simulink model "CTModel"  (R2021a)
settings: Solver=ode4  StartTime=0.0  StopTime=tstop  FixedStep=tstep  RelTol=1e-3
values from neighbouring files (symbols this model uses):
  ldotic = [-0.001; 0.005]    [data.m]
  Vmic = 1000    [data.m]
  xic = [15000; -30*d2r; 45*d2r; 10*d2r; 10*d2r; 20*d2r; 135*d2r]    [data.m]
settings Model: Creator=Ram Padmanabhan  LastModifiedBy=Ram Padmanabhan
settings DataIOCC: SaveOutput=off  SignalLogging=off  DSMLogging=off  SaveTime=off  ReturnWorkspaceOutputs=off
settings DebuggingCC: AlgebraicLoopMsg=none

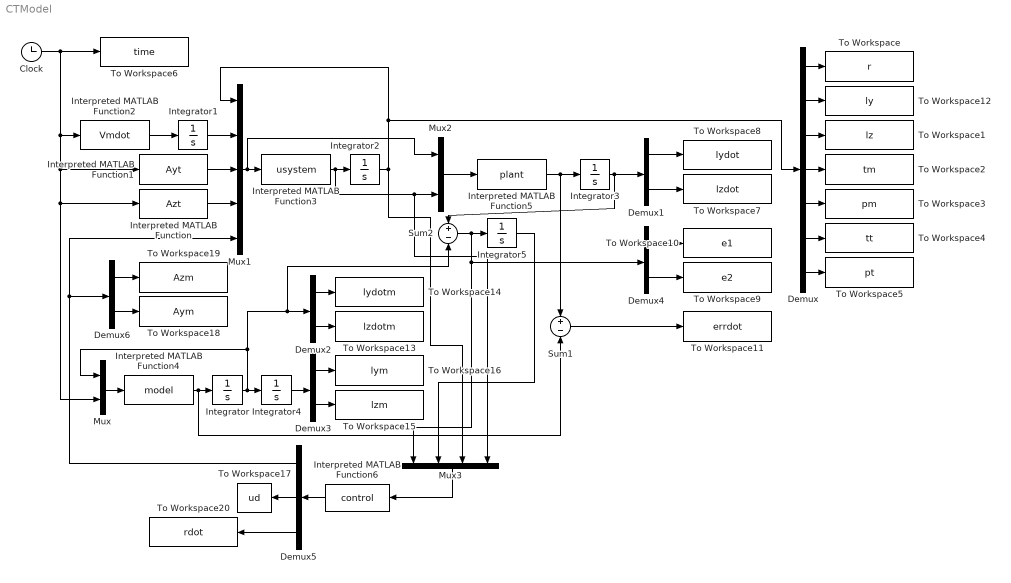
== system CTModel ==
  Clock : Clock
  Demux : Demux  Outputs=7
  Demux{1..4,6} (5 alike) : Demux  Outputs=2
  Demux5 : Demux  Outputs=3
  Integrator : Integrator
  Integrator1 : Integrator  InitialCondition=Vmic
  Integrator2 : Integrator  InitialCondition=xic
  Integrator3 : Integrator  InitialCondition=ldotic
  Integrator4 : Integrator
  Integrator5 : Integrator  InitialCondition=ldotic
  Interpreted MATLAB Function : MATLABFcn  MATLABFcn=Azt  OutputDimensions=1
  Interpreted MATLAB Function1 : MATLABFcn  MATLABFcn=Ayt  OutputDimensions=1
  Interpreted MATLAB Function2 : MATLABFcn  MATLABFcn=Vmdot  OutputDimensions=1
  Interpreted MATLAB Function3 : MATLABFcn  MATLABFcn=usystem  OutputDimensions=7
  Interpreted MATLAB Function4 : MATLABFcn  MATLABFcn=model  OutputDimensions=2
  Interpreted MATLAB Function5 : MATLABFcn  MATLABFcn=plant  OutputDimensions=2
  Interpreted MATLAB Function6 : MATLABFcn  MATLABFcn=control  OutputDimensions=5
  Mux : Mux  Inputs=2
  Mux1 : Mux  Inputs=5
  Mux2 : Mux  Inputs=2
  Mux3 : Mux
  Sum1 : Sum  Inputs=+|-
  Sum2 : Sum  Inputs=+|-
  To Workspace : ToWorkspace  VariableName=r  SampleTime=-1
  To Workspace1 : ToWorkspace  VariableName=lz  SampleTime=-1
  To Workspace10 : ToWorkspace  VariableName=e1  SampleTime=-1
  To Workspace11 : ToWorkspace  VariableName=errdot  SampleTime=-1
  To Workspace12 : ToWorkspace  VariableName=ly  SampleTime=-1
  To Workspace13 : ToWorkspace  VariableName=lzdotm  SampleTime=-1
  To Workspace14 : ToWorkspace  VariableName=lydotm  SampleTime=-1
  To Workspace15 : ToWorkspace  VariableName=lzm  SampleTime=-1
  To Workspace16 : ToWorkspace  VariableName=lym  SampleTime=-1
  To Workspace17 : ToWorkspace  VariableName=ud  SampleTime=-1
  To Workspace18 : ToWorkspace  VariableName=Aym  SampleTime=-1
  To Workspace19 : ToWorkspace  VariableName=Azm  SampleTime=-1
  To Workspace2 : ToWorkspace  VariableName=tm  SampleTime=-1
  To Workspace20 : ToWorkspace  VariableName=rdot  SampleTime=-1
  To Workspace3 : ToWorkspace  VariableName=pm  SampleTime=-1
  To Workspace4 : ToWorkspace  VariableName=tt  SampleTime=-1
  To Workspace5 : ToWorkspace  VariableName=pt  SampleTime=-1
  To Workspace6 : ToWorkspace  VariableName=time  SampleTime=-1
  To Workspace7 : ToWorkspace  VariableName=lzdot  SampleTime=-1
  To Workspace8 : ToWorkspace  VariableName=lydot  SampleTime=-1
  To Workspace9 : ToWorkspace  VariableName=e2  SampleTime=-1
  wires:
  Interpreted MATLAB Function3/1 -> Mux3/4, Mux2/2, Integrator2/1
  Mux1/1 -> Mux2/1, Interpreted MATLAB Function3/1
  Integrator2/1 -> Demux/1, Mux1/1, Mux3/3
  Interpreted MATLAB Function1/1 -> Mux1/3
  Interpreted MATLAB Function/1 -> Mux1/4
  Demux/1 -> To Workspace/1
  Demux/2 -> To Workspace12/1
  Demux/3 -> To Workspace1/1
  Demux/4 -> To Workspace2/1
  Demux/5 -> To Workspace3/1
  Demux/6 -> To Workspace4/1
  Demux/7 -> To Workspace5/1
  Clock/1 -> To Workspace6/1, Mux/2, Interpreted MATLAB Function/1, Interpreted MATLAB Function1/1, Interpreted MATLAB Function2/1
  Interpreted MATLAB Function2/1 -> Integrator1/1
  Integrator1/1 -> Mux1/2
  Interpreted MATLAB Function4/1 -> Sum1/2, Integrator/1
  Mux/1 -> Interpreted MATLAB Function4/1
  Mux2/1 -> Interpreted MATLAB Function5/1
  Interpreted MATLAB Function5/1 -> Integrator3/1, Sum1/1
  Integrator3/1 -> Sum2/1, Demux1/1
  Demux1/1 -> To Workspace8/1
  Demux1/2 -> To Workspace7/1
  Integrator/1 -> Sum2/2, Demux2/1, Mux/1, Integrator4/1
  Demux2/1 -> To Workspace14/1
  Demux2/2 -> To Workspace13/1
  Demux3/2 -> To Workspace15/1
  Demux3/1 -> To Workspace16/1
  Integrator4/1 -> Demux3/1
  Demux4/1 -> To Workspace10/1
  Demux4/2 -> To Workspace9/1
  Sum2/1 -> Integrator5/1, Mux3/1, Demux4/1
  Sum1/1 -> To Workspace11/1
  Mux3/1 -> Interpreted MATLAB Function6/1
  Integrator5/1 -> Mux3/2
  Interpreted MATLAB Function6/1 -> Demux5/1
  Demux5/2 -> To Workspace17/1
  Demux5/1 -> Mux1/5, Demux6/1
  Demux6/1 -> To Workspace19/1
  Demux6/2 -> To Workspace18/1
  Demux5/3 -> To Workspace20/1
